simulink model "eqprop_discrete"  (R2024b)
settings: Solver=VariableStepAuto  StartTime=0.0  StopTime=100  RelTol=1e-3
settings Model: Creator=merlin  LastModifiedBy=merlin

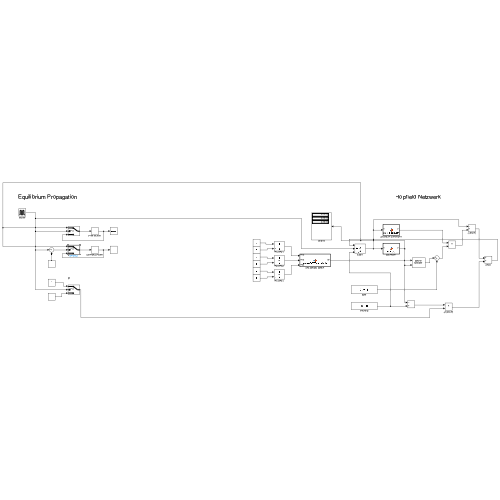
[thumbnail: Simulink's stored preview of the top-level diagram]
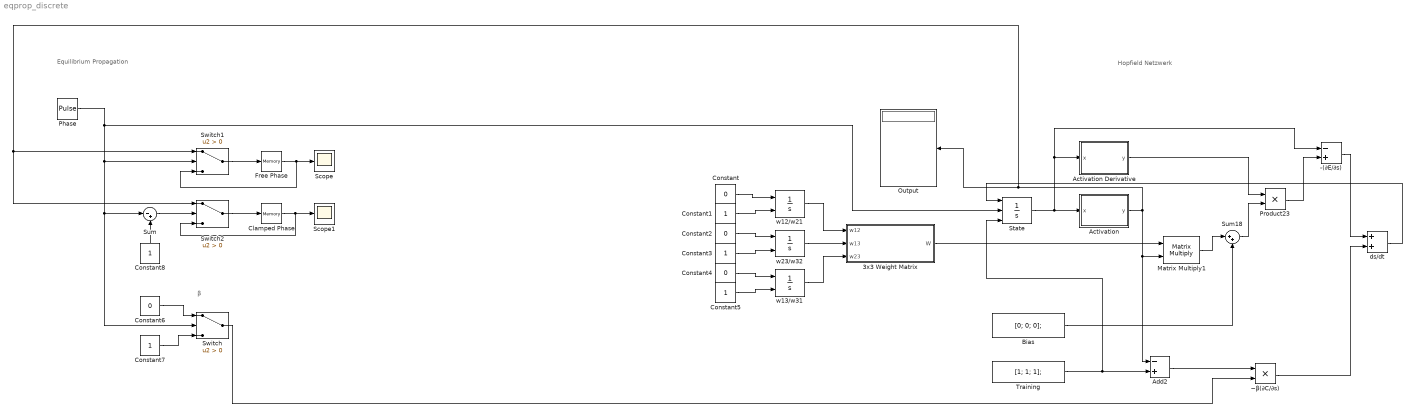
== system eqprop_discrete ==
  note: β
  note: Hopfield Netzwerk
  note: Equilibrium Propagation
  -(∂E/∂s) : Sum  Inputs=-+
  3x3 Weight Matrix : MATLAB Function  TreatAsAtomicUnit=on
  Activation : MATLAB Function  TreatAsAtomicUnit=on
  Activation Derivative : MATLAB Function  TreatAsAtomicUnit=on
  Add2 : Sum  Inputs=-+
  Bias : Constant  Value=[0; 0; 0];  VectorParams1D=off
  Clamped Phase : Memory
  Constant{,2,4,6} (4 alike) : Constant  Value=0
  Constant{1,3,5,7..8} (5 alike) : Constant
  Free Phase : Memory
  Matrix Multiply1 : Product  Multiplication=Matrix(*)
  Output : Display
  Phase : DiscretePulseGenerator  PulseType=Time based  Period=20  PulseWidth=50
  Product23 : Product
  Scope : Scope
  Scope1 : Scope
  State : Integrator  ExternalReset=either  InitialConditionSource=external
  Sum : Sum  Inputs=|-+
  Sum18 : Sum  Inputs=|++
  Switch : Switch  Criteria=u2 > Threshold  SaturateOnIntegerOverflow=off  InputSameDT=off
  Switch1 : Switch  Criteria=u2 > Threshold  SaturateOnIntegerOverflow=off  InputSameDT=off
  Switch2 : Switch  Criteria=u2 > Threshold  SaturateOnIntegerOverflow=off  InputSameDT=off
  Training : Constant  Value=[1; 1; 1];  VectorParams1D=off
  ds/dt : Sum
  w12/w21 : Integrator  InitialConditionSource=external
  w13/w31 : Integrator  InitialConditionSource=external
  w23/w32 : Integrator  InitialConditionSource=external
  −β(∂C/∂s) : Product
  wires:
  State/1 -> -(∂E/∂s)/1, Activation Derivative/1(x), Activation/1(x)
  Activation Derivative/1(y) -> Product23/1
  Matrix Multiply1/1 -> Sum18/1
  w23/w32/1 -> 3x3 Weight Matrix/2(w13)
  Training/1 -> State/3, Add2/2
  Bias/1 -> Sum18/2
  ds/dt/1 -> State/1
  Constant5/1 -> w13/w31/2
  w13/w31/1 -> 3x3 Weight Matrix/3(w23)
  Activation/1(y) -> Matrix Multiply1/2, Add2/1, Switch2/1, Switch1/1, Output/1
  -(∂E/∂s)/1 -> ds/dt/1
  −β(∂C/∂s)/1 -> ds/dt/2
  Add2/1 -> −β(∂C/∂s)/1
  Product23/1 -> -(∂E/∂s)/2
  Sum18/1 -> Product23/2
  w12/w21/1 -> 3x3 Weight Matrix/1(w12)
  Constant4/1 -> w13/w31/1
  Constant3/1 -> w23/w32/2
  Constant1/1 -> w12/w21/2
  Constant2/1 -> w23/w32/1
  Constant/1 -> w12/w21/1
  3x3 Weight Matrix/1(W) -> Matrix Multiply1/1
  Constant6/1 -> Switch/1
  Constant7/1 -> Switch/3
  Phase/1 -> State/2, Switch1/2, Sum/1, Switch/2
  Constant8/1 -> Sum/2
  Sum/1 -> Switch2/2
  Switch/1 -> −β(∂C/∂s)/2
  Switch1/1 -> Free Phase/1
  Switch2/1 -> Clamped Phase/1
  Free Phase/1 -> Switch1/3, Scope/1
  Clamped Phase/1 -> Switch2/3, Scope1/1

== matlab function eqprop_discrete/Activation Derivative ==
  data: x input; y output
function y = sigmoid_derivative(x)
sigmoid = 1 ./ (1 + exp(-x));
y = sigmoid .* (1 - sigmoid);
end

== matlab function eqprop_discrete/Activation ==
  data: x input; y output
function y = sigmoid(x)
y = 1 ./ (1 + exp(-x));
end

== matlab function eqprop_discrete/3x3 Weight Matrix ==
  data: w12 input; W output; w13 input; w23 input
function W = create3x3WeightMatrix(w12, w13, w23)
    W = [0,    w12,  w13;
         w12,  0,    w23;
         w13,  w23,  0];
end
